simulink model "Q4_nonlinear"  (R2021b)
settings: Solver=VariableStepAuto  StartTime=0.0  StopTime=100.0  RelTol=1e-3
undefined symbols (not defined in the file): K_statefeedback
settings Model: Creator=Sepehr Ahmadian  LastModifiedBy=sadeg
settings SolverCC: AlgebraicLoopSolver=TrustRegion
settings DebuggingCC: SFMachineParentedDataDiag=warning
settings SFSimCC: CustomCodeUndefinedFunction=UseInterfaceOnly

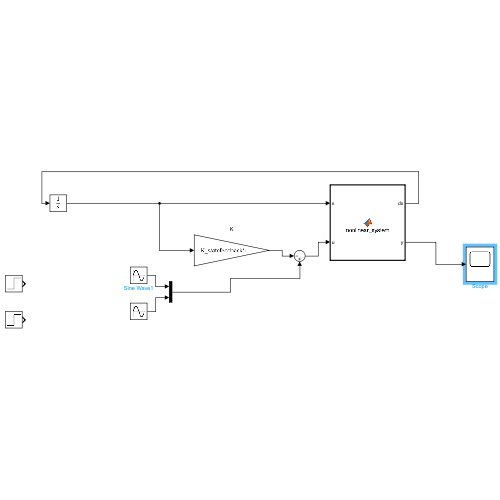
[thumbnail: Simulink's stored preview of the top-level diagram]
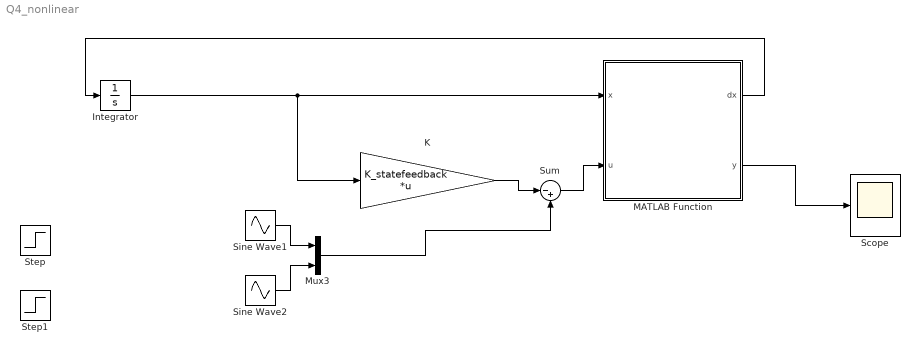
== system Q4_nonlinear ==
  Integrator : Integrator  InitialCondition=zeros(8,1)
  K : Gain  Gain=K_statefeedback  Multiplication=Matrix(K*u)
  MATLAB Function : MATLAB Function  TreatAsAtomicUnit=on
  Mux3 : Mux  Inputs=2
  Scope : Scope
  Sine Wave1 : Sin  Frequency=4  SampleTime=0
  Sine Wave2 : Sin  Frequency=4  SampleTime=0
  Step : Step  SampleTime=0
  Step1 : Step  SampleTime=0
  Sum : Sum  Inputs=|-+
  wires:
  Mux3/1 -> Sum/2
  Sine Wave2/1 -> Mux3/2
  Sine Wave1/1 -> Mux3/1
  MATLAB Function/1(dx) -> Integrator/1
  K/1 -> Sum/1
  Sum/1 -> MATLAB Function/2(u)
  Integrator/1 -> K/1, MATLAB Function/1(x)
  MATLAB Function/2(y) -> Scope/1

== matlab function Q4_nonlinear/MATLAB Function ==
  data: x input size=8; u input size=2; dx output size=8; y output size=2
function [dx, y] = nonlinear_system(x, u)

    x = reshape(x, [], 1);
    assert(length(x) == 8, 'Input x must be a vector of size 8.');


    mb = 0.11;  % mass of ball (kg)
    Jb = 1.76e-5;  % rotational moment of inertia of the ball (kgm^2)
    Rb = 0.02;  % radius of the ball (m)
    g = 9.8;  % acceleration due to gravity (m/s^2)

    % B_parameter
    B_parameter = mb / (mb + (Jb / Rb^2));

    B = [0, 0; 
         0, 0; 
         0, 0; 
         1, 0; 
         0, 0; 
         0, 0; 
         0, 0; 
         0, 1];  % 8x2 matrix

    % Nonlinear dynamics equations
    dx1 = x(2);
    dx2 = B_parameter * (x(1) * x(4)^2 + x(4) * x(5) * x(8) - g * sin(x(3))) %+ B(4, :) * u;  % Input influence on dx2
    dx3 = x(4);
    dx4 = 0;

    dx5 = x(6);
    dx6 = B_parameter * (x(5) * x(8)^2 + x(1) * x(4) * x(8) - g * sin(x(7))) %+ B(8, :) * u;  % Input influence on dx6
    dx7 = x(8);
    dx8 = 0;

    % State derivative
    dx = [dx1; dx2; dx3; dx4; dx5; dx6; dx7; dx8]+ B*u;

    % Output equation: y = C*x
    C = [1, 0, 0, 0, 0, 0, 0, 0; 
         0, 0, 0, 0, 1, 0, 0, 0];  % C matrix (2x8)

    y = C * x;  % Compute the outputs
end
